simulink model "cluth"  (R2024b)
settings: Solver=VariableStepAuto  StartTime=0.0  StopTime=10.0  RelTol=1e-3
values from neighbouring files (symbols this model uses):
  fk = 4000    [parameters.m]
  I1 = 1    [parameters.m]
  I2 = 5    [parameters.m]
  mu = 0.3    [parameters.m]
  ra = 0.15    [parameters.m]
  ri = 0.1    [parameters.m]
  T1 = 200    [parameters.m]
  x2 = 200    [parameters.m]
  x4 = 0    [parameters.m]
settings Model: Creator=kavin  LastModifiedBy=kavin

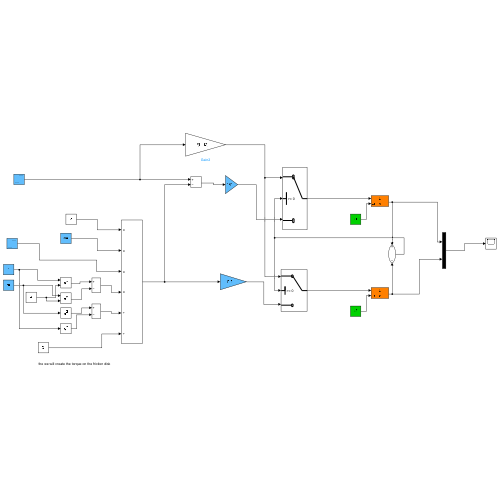
[thumbnail: Simulink's stored preview of the top-level diagram]
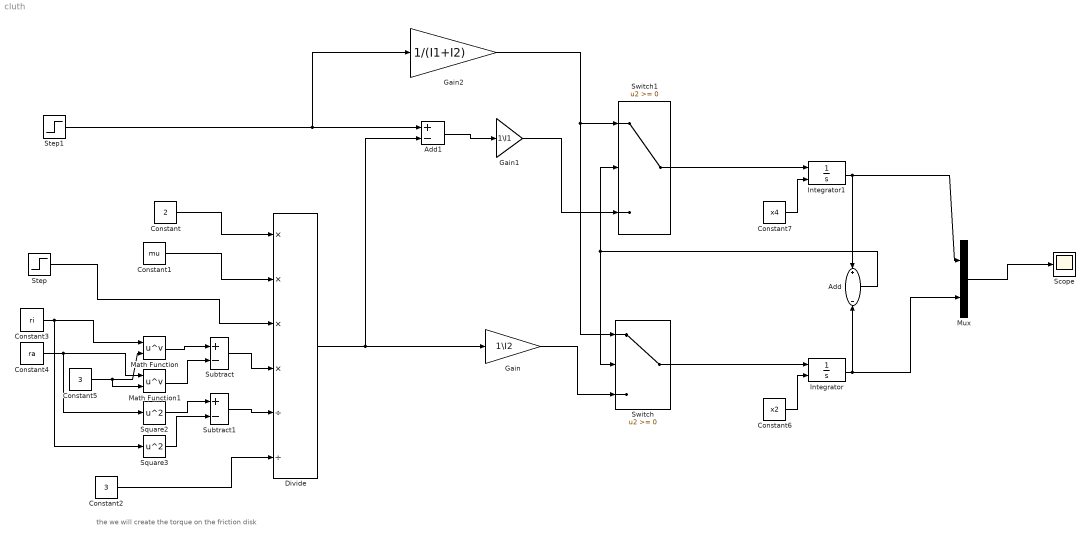
== system cluth ==
  note: the we will create the torque on the friction disk
  Add : Sum  Inputs=+-
  Add1 : Sum  Inputs=+-
  Constant : Constant  Value=2
  Constant1 : Constant  Value=mu
  Constant2 : Constant  Value=3
  Constant3 : Constant  Value=ri
  Constant4 : Constant  Value=ra
  Constant5 : Constant  Value=3
  Constant6 : Constant  Value=x2
  Constant7 : Constant  Value=x4
  Divide : Product  Inputs=****//
  Gain : Gain  Gain=1\I2
  Gain1 : Gain  Gain=1\I1
  Gain2 : Gain  Gain=1/(I1+I2)
  Integrator : Integrator  InitialConditionSource=external
  Integrator1 : Integrator  InitialConditionSource=external
  Math Function : Math  Operator=pow
  Math Function1 : Math  Operator=pow
  Mux : Mux  Inputs=2
  Scope : Scope
  Square2 : Math  Operator=square
  Square3 : Math  Operator=square
  Step : Step  After=fk  SampleTime=0
  Step1 : Step  After=T1  SampleTime=0
  Subtract : Sum  Inputs=+-
  Subtract1 : Sum  Inputs=+-
  Switch : Switch  SaturateOnIntegerOverflow=off  InputSameDT=off
  Switch1 : Switch  SaturateOnIntegerOverflow=off  InputSameDT=off
  wires:
  Constant/1 -> Divide/1
  Constant1/1 -> Divide/2
  Step/1 -> Divide/3
  Constant2/1 -> Divide/6
  Constant3/1 -> Square3/1, Math Function/1
  Constant4/1 -> Square2/1, Math Function1/1
  Constant5/1 -> Math Function1/2, Math Function/2
  Math Function/1 -> Subtract/1
  Math Function1/1 -> Subtract/2
  Square2/1 -> Subtract1/1
  Square3/1 -> Subtract1/2
  Subtract/1 -> Divide/4
  Subtract1/1 -> Divide/5
  Switch/1 -> Integrator/1
  Constant6/1 -> Integrator/2
  Gain/1 -> Switch/3
  Switch1/1 -> Integrator1/1
  Constant7/1 -> Integrator1/2
  Add/1 -> Switch/2, Switch1/2
  Integrator1/1 -> Add/1, Mux/1
  Integrator/1 -> Mux/2, Add/2
  Step1/1 -> Gain2/1, Add1/1
  Divide/1 -> Add1/2, Gain/1
  Add1/1 -> Gain1/1
  Gain1/1 -> Switch1/3
  Gain2/1 -> Switch/1, Switch1/1
  Mux/1 -> Scope/1
